simulink model "AutomatedGuidedVehicleHybridControllerslx"  (R2017a)
settings: Solver=FixedStepAuto  StartTime=0.0  StopTime=100.0  FixedStep=0.001  RelTol=1e-3
libraries: simulink x1
settings Model: Creator=a01207112  LastModifiedBy=a01207112
settings SFSimCC: SFSimEcho=off  SimCtrlC=off

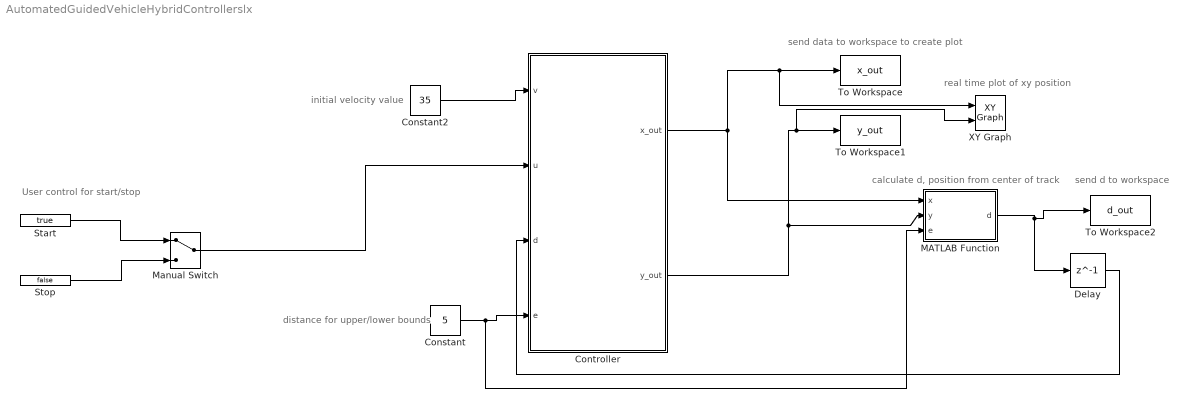
== system AutomatedGuidedVehicleHybridControllerslx ==
  note: send d to workspace
  note: calculate d, position from center of track
  note: real time plot of xy position
  note: send data to workspace to create plot
  note: initial velocity value
  note: distance for upper/lower bounds
  note: User control for start/stop
  Constant : Constant  Value=5
  Constant2 : Constant  Value=35
  Controller : Stateflow chart  TreatAsAtomicUnit=on
  Delay : Delay  DelayLength=1  InitialCondition=0
  MATLAB Function : MATLAB Function  TreatAsAtomicUnit=on
  Manual Switch : ManualSwitch
  Start : Constant  Value=true
  Stop : Constant  Value=false
  To Workspace : ToWorkspace  VariableName=x_out  SaveFormat=Timeseries  SampleTime=-1
  To Workspace1 : ToWorkspace  VariableName=y_out  SaveFormat=Timeseries  SampleTime=-1
  To Workspace2 : ToWorkspace  VariableName=d_out  SaveFormat=Timeseries  SampleTime=-1
  XY Graph : simulink/Sinks/XY Graph  xmin=-60  xmax=60  ymin=-60  ymax=60  st=-1
  wires:
  Manual Switch/1 -> Controller/2(u)
  Start/1 -> Manual Switch/1
  Stop/1 -> Manual Switch/2
  Controller/1(x_out) -> XY Graph/1, To Workspace/1, MATLAB Function/1(x)
  Controller/2(y_out) -> XY Graph/2, To Workspace1/1, MATLAB Function/2(y)
  Constant2/1 -> Controller/1(v)
  Delay/1 -> Controller/3(d)
  Constant/1 -> MATLAB Function/3(e), Controller/4(e)
  MATLAB Function/1(d) -> To Workspace2/1, Delay/1

== matlab function AutomatedGuidedVehicleHybridControllerslx/MATLAB Function ==
  data: x input; d output; y input; e input
function d = fcn(x,y,e)
%#codegen

%assert(-4<(sqrt(x^2+y^2)-50)<4,'Safety requirement violated: d=%d',(sqrt(x^2+y^2)-50));
%calculate distance d based on x and y position and radius of track
d = sqrt(x^2+y^2)-50;
%assert(-1.5*e<d<1.5*e,'Safety requirement violated: d=%d',d);


%safety requirement%
%car does not exceed allowable distance past upperbound
assert(d<1.5*e,'Safety requirement violated: d=%d',d);
%car does not exceed allowable distance past lowerbound
assert(d>-1.5*e,'Safety requirement violated: d=%d',d);

== stateflow chart AutomatedGuidedVehicleHybridControllerslx/Controller ==
  settings: updateMethod=CONTINUOUS
  state Straight%car going straight
    du:%during
    x_dot=(v*cos(theta));%time derivative x position
    y_dot=(v*sin(theta));%time derivative y position
    theta_dot=0;%time derivative angle
    x_out=x; %output x position
    y_out=y;%output y position
  state Right%car is turning right, slow down velocity
    du: %during
    x_dot=(v*cos(theta))/2;%time derivative x position
    y_dot=(v*sin(theta))/2;%time derivative y position
    theta_dot=-pi;%time derivative angle
    x_out=x;%output x position
    y_out=y;%output y position
  state Stop%car is stopped
    du: %during
    x_dot=0; %time derivative x position
    y_dot=0;%time derivative y position
    theta_dot=0;%time derivative angle
  state Left% car going left, slow down velocity
    du:%during
    x_dot=(v*cos(theta))/2;%time derivative x position
    y_dot=(v*sin(theta))/2;%time derivative y position
    theta_dot=pi;%time derivative angle
    x_out=x;%output x position
    y_out=y;%output y position
  Right%car is turning right, slow down velocity -> Right%car is turning right, slow down velocity [order 3] : [d>=e&u==true]%car passed upper bound
  Straight%car going straight -> Straight%car going straight [order 4] : [(-e<=d<=e) & u==true]%car within bounds
  Right%car is turning right, slow down velocity -> Straight%car going straight [order 2] : [d<=e]{theta=theta+(pi*0.01)}%reentered bounds
      | %adjust for accumulating error
  Straight%car going straight -> Right%car is turning right, slow down velocity [order 1] : [d>=e]%passed upper bound
  Straight%car going straight -> Stop%car is stopped [order 3] : [u==false]%user stop
  Stop%car is stopped -> Straight%car going straight [order 2] : [u==true & (-e<=d<=e)]%user start
      | %car within bounds
  Straight%car going straight -> Left% car going left, slow down velocity [order 2] : [d<=-e]%passed lower bound
  Left% car going left, slow down velocity -> Straight%car going straight [order 1] : [d>=-e]{theta=theta-(pi*0.01)}%car reentered bounds
      | %adjust for accumulating error
  Right%car is turning right, slow down velocity -> Stop%car is stopped [order 1] : [u==false]%user stop
  Stop%car is stopped -> Right%car is turning right, slow down velocity [order 1] : [u==true & d>=e]%user start
      | %car passed upper bound
  Stop%car is stopped -> Left% car going left, slow down velocity [order 3] : [u==true&d<=-e]
  Left% car going left, slow down velocity -> Stop%car is stopped [order 3] : [u==false]%user stop
  (default) -> Stop%car is stopped : {x=-30; y=35; theta=0.4*pi}%initial values
  Left% car going left, slow down velocity -> Left% car going left, slow down velocity [order 2] : [d<=-e & u==true]%car passed lower bound
  data: theta local; v input; u input boolean; d input double; e input double =5; y local; x local; x_out output =x0; y_out output =y0
  data theta settings: updateMethod=SF_CONTINUOUS_TIME_DATA
  data y settings: updateMethod=SF_CONTINUOUS_TIME_DATA
  data x settings: updateMethod=SF_CONTINUOUS_TIME_DATA
